simulink model "IEEE_9bus_1SG_1VSC_1DP_vol2"  (R2023b)
settings: Solver=ode8  StartTime=0.001  StopTime=60  RelTol=1e-4  EnableMultiTasking=on
PreLoadFcn:
  | ct = 1.083
values from neighbouring files (symbols this model uses):
  kp3 = 5    [main.m]
  Pmax3 = 1.15    [main.m]
  Pmin3 = 0.850    (= 0.85)    [main.m]
  Pnom = 100e6    (= 100000000)    [main.m]
  t_st = 5    [main.m]
  ts_pi = 5    [main.m]
  Vnom_prim = 230e3    (= 230000)    [main.m]
undefined symbols (not defined in the file or in its folder): D1, Delta
libraries: spsThreePhaseVIMeasurementLib x13, spsPLL3phLib x10, spsSequenceAnalyzerLib x10, spsLoadFlowBusLib x9, eeSinusoidalMeasurementV2 x9, spsThreePhasePISectionLineLib x6, slpidlib x6, jailib x4, spsPowerPositiveSequenceLib x4, spsThreePhaseTransformerTwoWindingsLib x3, spsMeanLib x3, spsDCVoltageSourceLib x2
(part 1 of 2)
settings Model: Creator=jp536285  LastModifiedBy=Administrator
settings SolverCC: AlgebraicLoopSolver=TrustRegion  AutoInsertRateTranBlk=on
settings DataIOCC: FinalStateName=xFinal_no_ex_vol2  InitialState=xFinal_no_ex_vol2  LoadInitialState=on  SaveOperatingPoint=on  SaveFormat=Array  SaveOutput=off  SaveTime=off  ReturnWorkspaceOutputs=off
settings OptimizationCC: LifeSpan=inf
settings DebuggingCC: UnderspecifiedInitializationDetection=Classic  MergeDetectMultiDrivingBlocksExec=none  SolverPrmCheckMsg=warning  StateNameClashWarn=warning  SFUnexpectedBacktrackingDiag=warning  SFNoUnconditionalDefaultTransitionDiag=warning  SFExecutionAtInitializationDiag=none  ArithmeticOperatorsInVariantConditions=warning
settings HardwareCC: ProdBitPerPointer=32  ProdBitPerSizeT=32  ProdBitPerPtrDiffT=32  ProdLargestAtomicFloat=None  ProdIntDivRoundTo=Undefined  ProdEndianess=Unspecified  ProdWordSize=32  ProdHWDeviceType=32-bit Generic
settings ModelReferenceCC: PropagateSignalLabelsOutOfModel=off
settings SFSimCC: SimUseLocalCustomCode=off  CustomCodeUndefinedFunction=UseInterfaceOnly
settings RTWCC: RTWUseLocalCustomCode=off
settings CodeAppCC: StateflowObjectComments=on
settings GRTTargetCC: TargetLangStandard=C89/C90 (ANSI)
settings ConfigComp: CovMetricSettings=dw  CovSaveCumulativeToWorkspaceVar=on  CovSaveSingleToWorkspaceVar=on  CovExternalEMLEnable=off
settings SimscapeCC: SimscapeNormalizeSystem=off

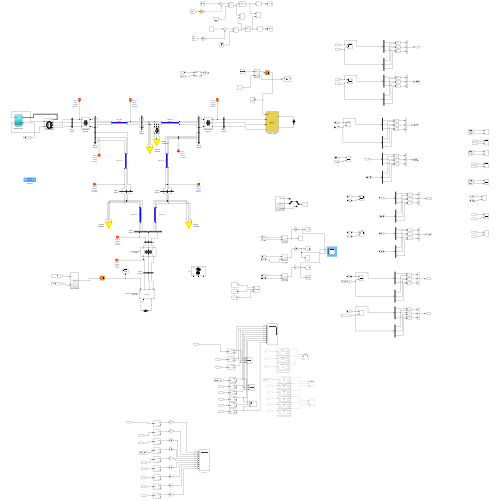
[thumbnail: Simulink's stored preview of the top-level diagram]
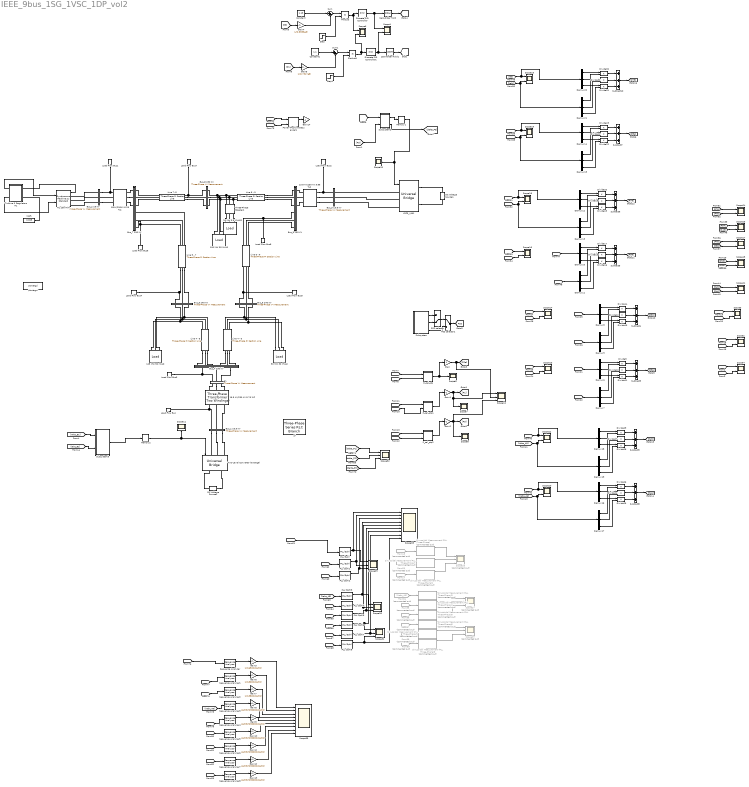
== system IEEE_9bus_1SG_1VSC_1DP_vol2 ==
  " Line 4 - 6" : spsThreePhasePISectionLineLib/Three-Phase PI Section Line  LConnTagsString=a|b|c  RConnTagsString=A|B|C  Length=100  Frequency=60  Resistances=[ 0.08993 0.224825]  Inductances="[ 1.29e-3  3.22e-3]"  Capacitances=[7.922e-9 4.74e-9]  mask(Three-Phase PI Section Line){}
      mask Display:
      | % This is a new mask on top of the base mask.
      | % Use "View base mask" link below to see the base mask.
      | patch([0.0 0.0 1 1 0.0 0.0 ],[0.4 0.7 0.7 0.4 0.4 0.7],[0 0 1]);
      | patch([0.4 0.4 0.42 0.42],[0.4 0.75 0.75 0.4],[1 0 0]);
      | patch([0.38 0.38 0.57 0.57],[0.7 0.75 0.75 0.7],[1 0 0]);
      | patch([0.53 0.53 0.55 0.55],[0.4 0.75 0.75 0.4],[1 0 0]);
  " Line 6 - 9" : spsThreePhasePISectionLineLib/Three-Phase PI Section Line  LConnTagsString=a|b|c  RConnTagsString=A|B|C  Length=100  Frequency=60  Resistances=[ 0.20631 0.5157]  Inductances="[ 2.38e-3  6.09e-3]"  Capacitances=[17.95e-9 10.55e-9]  mask(Three-Phase PI Section Line){}
      mask Display:
      | % This is a new mask on top of the base mask.
      | % Use "View base mask" link below to see the base mask.
      | patch([0.0 0.0 1 1 0.0 0.0 ],[0.4 0.7 0.7 0.4 0.4 0.7],[0 0 1]);
      | patch([0.4 0.4 0.42 0.42],[0.4 0.75 0.75 0.4],[1 0 0]);
      | patch([0.38 0.38 0.57 0.57],[0.7 0.75 0.75 0.7],[1 0 0]);
      | patch([0.53 0.53 0.55 0.55],[0.4 0.75 0.75 0.4],[1 0 0]);
  100 MW 35 MVAR : jailib/Load  SystemSampleTime=-1  VariantActivationTime=update diagram  AllowFlexibleInterface=on  Latency=0  AutoFrameSizeCalculation=off
      link override Three-Phase Parallel RLC Load: NominalVoltage=(230000)*1.01602  ActivePower=100e6  InductivePower=35e6  LoadType=constant PQ
      settings: SourceProductName=Power Library
  125 MW 50 MVAR : jailib/Load  SystemSampleTime=-1  VariantActivationTime=update diagram  AllowFlexibleInterface=on  Latency=0  AutoFrameSizeCalculation=off
      link override Three-Phase Parallel RLC Load: NominalVoltage=(230000)*0.996183  ActivePower=125e6  InductivePower=50e6  LoadType=constant PQ
      settings: SourceProductName=Power Library
  13.8 KV/230 KV 5.86 %Z : spsThreePhaseTransformerTwoWindingsLib/Three-Phase Transformer (Two Windings)  Winding1Connection=Delta (D1)  Winding2Connection=Yg  CoreType=Three single-phase transformers  SetSaturation=off  Hysteresis=off  DataFile='hysteresis'  SetInitialFlux=off  Measurements=None  UNITS=pu  NominalPower=[ 100e6 , 60 ]  Winding1=[ 13.8e3 , 1e-6 , 0 ]  Winding2=[ 230e3 , 1e-6, 0.0586 ]  Rm=500  Lm=500  L0=0.5  Saturation=[ 0,0 ; 0.0024,1.2 ; 1.0,1.52 ]  InitialFluxes=[ 0.8 , -0.8 , 0.7 ]  BreakLoop=off  DiscreteSolver=Trapezoidal iterative  DataType=off  TransfoNumber=1
  "16.5 KV/230 KV 5.76 %Z     " : spsThreePhaseTransformerTwoWindingsLib/Three-Phase Transformer (Two Windings)  Winding1Connection=Delta (D1)  Winding2Connection=Yg  CoreType=Three single-phase transformers  SetSaturation=off  Hysteresis=off  DataFile='hysteresis'  SetInitialFlux=off  Measurements=None  UNITS=pu  NominalPower=[ 100e6 , 60 ]  Winding1=[ 16.5e3 , 1e-6, 0 ]  Winding2=[ 230e3 ,1e-6, 0.0576 ]  Rm=500  Lm=500  L0=0.5  Saturation=[ 0,0 ; 0.0024,1.2 ; 1.0,1.52 ]  InitialFluxes=[ 0.8 , -0.8 , 0.7 ]  BreakLoop=off  DiscreteSolver=Trapezoidal iterative  DataType=off  TransfoNumber=1
  18KV/230KV 6.25 %Z : spsThreePhaseTransformerTwoWindingsLib/Three-Phase Transformer (Two Windings)  Winding1Connection=Delta (D1)  Winding2Connection=Yg  CoreType=Three single-phase transformers  SetSaturation=off  Hysteresis=off  DataFile='hysteresis'  SetInitialFlux=off  Measurements=None  UNITS=pu  NominalPower=[ 100e6 , 60 ]  Winding1=[ 18e3 , 1e-6 , 0]  Winding2=[ 230e3 , 1e-6, 0.0625 ]  Rm=500  Lm=500  L0=0.5  Saturation=[ 0,0 ; 0.0024,1.2 ; 1.0,1.52 ]  InitialFluxes=[ 0.8 , -0.8 , 0.7 ]  BreakLoop=off  DiscreteSolver=Trapezoidal iterative  DataType=off  TransfoNumber=1
  20 MW 3.5 MVAR2 : jailib/Load  SystemSampleTime=-1  VariantActivationTime=update diagram  AllowFlexibleInterface=on  Latency=0  AutoFrameSizeCalculation=off
      link override Three-Phase Parallel RLC Load: NominalVoltage=(230000)*1.01602  ActivePower=10e6  InductivePower=0  LoadType=constant PQ
      settings: SourceProductName=Power Library
  90 MW 30 MVAR : jailib/Load  SystemSampleTime=-1  VariantActivationTime=update diagram  AllowFlexibleInterface=on  Latency=0  AutoFrameSizeCalculation=off
      link override Three-Phase Parallel RLC Load: NominalVoltage=(230000)*1.01315  ActivePower=90e6  InductivePower=30e6  LoadType=constant PQ
      settings: SourceProductName=Power Library
  B1 : spsThreePhaseVIMeasurementLib/Three-Phase V-I Measurement  VoltageMeasurement=phase-to-ground  SetLabelV=on  LabelV=Vabc_B1  Vpu=off  VpuLL=off  CurrentMeasurement=yes  SetLabelI=on  LabelI=Iabc_B1  Ipu=off  Pbase=100e6  Vbase=500e3  OutputType=Magnitude  PhasorSimulation=off  PSBequivalent=0
  Bus_1 16.5 KV : spsThreePhaseVIMeasurementLib/Three-Phase V-I Measurement  VoltageMeasurement=phase-to-phase  SetLabelV=on  LabelV=Vabc_1  Vpu=off  VpuLL=off  CurrentMeasurement=yes  SetLabelI=on  LabelI=Iabc_1  Ipu=off  Pbase=100e6  Vbase=16.5e3  OutputType=Complex  PhasorSimulation=off  PSBequivalent=0
  Bus_2 18 KV : spsThreePhaseVIMeasurementLib/Three-Phase V-I Measurement  VoltageMeasurement=phase-to-phase  SetLabelV=on  LabelV=Vabc_2  Vpu=off  VpuLL=off  CurrentMeasurement=yes  SetLabelI=on  LabelI=Iabc_2  Ipu=off  Pbase=100e6  Vbase=18e3  OutputType=Complex  PhasorSimulation=off  PSBequivalent=0
  Bus_3 13.8 KV : spsThreePhaseVIMeasurementLib/Three-Phase V-I Measurement  VoltageMeasurement=phase-to-phase  SetLabelV=on  LabelV=Vabc_3  Vpu=off  VpuLL=off  CurrentMeasurement=yes  SetLabelI=on  LabelI=Iabc_3  Ipu=off  Pbase=100e6  Vbase=13.8e3  OutputType=Complex  PhasorSimulation=off  PSBequivalent=0
  Bus_4 230 KV : Subsystem
  Bus_5 230 KV : spsThreePhaseVIMeasurementLib/Three-Phase V-I Measurement  VoltageMeasurement=phase-to-ground  SetLabelV=on  LabelV=Vabc_5  Vpu=off  VpuLL=off  CurrentMeasurement=yes  SetLabelI=on  LabelI=Iabc_5  Ipu=off  Pbase=100e6  Vbase=230e3  OutputType=Complex  PhasorSimulation=off  PSBequivalent=0
  Bus_6 230 KV : spsThreePhaseVIMeasurementLib/Three-Phase V-I Measurement  VoltageMeasurement=phase-to-ground  SetLabelV=on  LabelV=Vabc_6  Vpu=off  VpuLL=off  CurrentMeasurement=yes  SetLabelI=on  LabelI=Iabc_6  Ipu=off  Pbase=100e6  Vbase=230e3  OutputType=Complex  PhasorSimulation=off  PSBequivalent=0
  Bus_7 230 KV : Subsystem
  Bus_8 230 KV : spsThreePhaseVIMeasurementLib/Three-Phase V-I Measurement  VoltageMeasurement=phase-to-ground  SetLabelV=on  LabelV=Vabc_8  Vpu=off  VpuLL=off  CurrentMeasurement=yes  SetLabelI=on  LabelI=Iabc_8  Ipu=off  Pbase=100e6  Vbase=230e3  OutputType=Complex  PhasorSimulation=off  PSBequivalent=0
  Bus_9 230 KV : Subsystem
  Constant : Constant  Value=1.13
  Constant1 : Constant  Value=1.1
  DC Voltage Source1 : spsDCVoltageSourceLib/DC Voltage Source  Amplitude=2*13.8e3  Measurements=None
  DC Voltage Source2 : spsDCVoltageSourceLib/DC Voltage Source  Amplitude=2*16.5e3  Measurements=None
  Demux{6..21} (16 alike) : Demux  Outputs=3
  Discrete PID Controller : slpidlib/PID Controller  Controller=PI  Form=Parallel  TimeDomain=Discrete-time  UseExternalTs=off  SampleTime=-1  IntegratorMethod=Forward Euler  FilterMethod=Forward Euler  ControllerParametersSource=internal  P=0.001  I=0.015  UseKiTs=off  D=0  N=100  UseFilter=on  TunerSelectOption=Transfer Function Based (PID Tuner App)  InitialConditionSource=internal  InitialConditionForIntegrator=0  InitialConditionForFilter=0  DifferentiatorICPrevScaledInput=0  ExternalReset=none  TrackingMode=off  Kt=1  LimitOutput=off  SatLimitsSource=internal  UpperSaturationLimit=inf  LowerSaturationLimit=-inf  LinearizeAsGain=off  AntiWindupMode=none  Kb=1  LimitIntegrator=off  UpperIntegratorSaturationLimit=inf  LowerIntegratorSaturationLimit=-inf  POutMin=[]  POutMax=[]  IOutMin=[]  IOutMax=[]  DOutMin=[]  DOutMax=[]  NOutMin=[]  NOutMax=[]  SumOutMin=[]  SumOutMax=[]  SaturationOutMin=[]  SaturationOutMax=[]  PParamMin=[]  PParamMax=[]  IParamMin=[]  IParamMax=[]  DParamMin=[]  DParamMax=[]  NParamMin=[]  NParamMax=[]  KbParamMin=[]  KbParamMax=[]  KtParamMin=[]  KtParamMax=[]  KbOutMin=[]  KbOutMax=[]  KtOutMin=[]  KtOutMax=[]  IntegratorOutMin=[]  IntegratorOutMax=[]  FilterOutMin=[]  FilterOutMax=[]  SumI1OutMin=[]  SumI1OutMax=[]  SumI2OutMin=[]  SumI2OutMax=[]  SumI3OutMin=[]  SumI3OutMax=[]  SumI4OutMin=[]  SumI4OutMax=[]  SumDOutMin=[]  SumDOutMax=[]  DifferentiatorOutMin=[]  DifferentiatorOutMax=[]  FilterDiffOutCoefMin=[]  FilterDiffOutCoefMax=[]  ReciprocalOutMin=[]  ReciprocalOutMax=[]  SumDenOutMin=[]  SumDenOutMax=[]  SumNumOutMin=[]  SumNumOutMax=[]  DivideOutMin=[]  DivideOutMax=[]  UdiffTsProdOutMin=[]  UdiffTsProdOutMax=[]  NTsProdOutMin=[]  NTsProdOutMax=[]  UintegralTsProdOutMin=[]  UintegralTsProdOutMax=[]  UngainTsProdOutMin=[]  UngainTsProdOutMax=[]  ClampingZeroOutDataTypeStr=Inherit: Inherit via back propagation  ClampingZeroOutMin=[]  ClampingZeroOutMax=[]  FilterDenConstantOutDataTypeStr=Inherit: Inherit via back propagation  FilterDenConstantOutMin=[]  FilterDenConstantOutMax=[]  PCopyOutDataTypeStr=Inherit: Inherit via back propagation  PCopyOutMin=[]  PCopyOutMax=[]  NCopyOutDataTypeStr=Inherit: Inherit via back propagation  NCopyOutMin=[]  NCopyOutMax=[]  IntegratorContinuousStateAttributes=''  IntegratorStateMustResolveToSignalObject=off  IntegratorRTWStateStorageClass=Auto  FilterContinuousStateAttributes=''  FilterStateMustResolveToSignalObject=off  FilterRTWStateStorageClass=Auto  ParallelPVariant=InternalParameters  IdealPVariant=Disabled  IVariant=InternalParameters  DVariant=Disabled  IntegratorVariant=Discrete  SatVariant=Disabled  AWVariant=Passthrough  PCopyVariant=Disabled  TRVariant=Disabled  FdbkBlocksVariant=Forward  IdealPFdbkVariant=Disabled  SatFdbkVariant=Disabled  DerivativeFilterVariant=Disabled  NVariant=Disabled  NCopyVariant=Disabled_SignalSpec  FilterICVariant=Disabled  IntegratorICVariant=InternalICs  ExternalResetVariant=Disabled  TRSumVariant=Passthrough  SumFdbkVariant=Disabled  SumVariant=Sum_PI  TsampFilterVariant=InternalTs  TsampNgainVariant=Passthrough  TsampIntegralVariant=Disabled_SignalSpec  ExternalSaturationOutDataTypeStr=Inherit: Same as second input
      settings: LibrarySourceBlock=simulink/Discrete/Discrete PID Controller
  Discrete PID Controller1 : slpidlib/PID Controller  Controller=PI  Form=Parallel  TimeDomain=Discrete-time  UseExternalTs=off  SampleTime=-1  IntegratorMethod=Forward Euler  FilterMethod=Forward Euler  ControllerParametersSource=internal  P=0.001  I=0.015  UseKiTs=off  D=0  N=100  UseFilter=on  TunerSelectOption=Transfer Function Based (PID Tuner App)  InitialConditionSource=internal  InitialConditionForIntegrator=0  InitialConditionForFilter=0  DifferentiatorICPrevScaledInput=0  ExternalReset=none  TrackingMode=off  Kt=1  LimitOutput=off  SatLimitsSource=internal  UpperSaturationLimit=inf  LowerSaturationLimit=-inf  LinearizeAsGain=off  AntiWindupMode=none  Kb=1  LimitIntegrator=off  UpperIntegratorSaturationLimit=inf  LowerIntegratorSaturationLimit=-inf  POutMin=[]  POutMax=[]  IOutMin=[]  IOutMax=[]  DOutMin=[]  DOutMax=[]  NOutMin=[]  NOutMax=[]  SumOutMin=[]  SumOutMax=[]  SaturationOutMin=[]  SaturationOutMax=[]  PParamMin=[]  PParamMax=[]  IParamMin=[]  IParamMax=[]  DParamMin=[]  DParamMax=[]  NParamMin=[]  NParamMax=[]  KbParamMin=[]  KbParamMax=[]  KtParamMin=[]  KtParamMax=[]  KbOutMin=[]  KbOutMax=[]  KtOutMin=[]  KtOutMax=[]  IntegratorOutMin=[]  IntegratorOutMax=[]  FilterOutMin=[]  FilterOutMax=[]  SumI1OutMin=[]  SumI1OutMax=[]  SumI2OutMin=[]  SumI2OutMax=[]  SumI3OutMin=[]  SumI3OutMax=[]  SumI4OutMin=[]  SumI4OutMax=[]  SumDOutMin=[]  SumDOutMax=[]  DifferentiatorOutMin=[]  DifferentiatorOutMax=[]  FilterDiffOutCoefMin=[]  FilterDiffOutCoefMax=[]  ReciprocalOutMin=[]  ReciprocalOutMax=[]  SumDenOutMin=[]  SumDenOutMax=[]  SumNumOutMin=[]  SumNumOutMax=[]  DivideOutMin=[]  DivideOutMax=[]  UdiffTsProdOutMin=[]  UdiffTsProdOutMax=[]  NTsProdOutMin=[]  NTsProdOutMax=[]  UintegralTsProdOutMin=[]  UintegralTsProdOutMax=[]  UngainTsProdOutMin=[]  UngainTsProdOutMax=[]  ClampingZeroOutDataTypeStr=Inherit: Inherit via back propagation  ClampingZeroOutMin=[]  ClampingZeroOutMax=[]  FilterDenConstantOutDataTypeStr=Inherit: Inherit via back propagation  FilterDenConstantOutMin=[]  FilterDenConstantOutMax=[]  PCopyOutDataTypeStr=Inherit: Inherit via back propagation  PCopyOutMin=[]  PCopyOutMax=[]  NCopyOutDataTypeStr=Inherit: Inherit via back propagation  NCopyOutMin=[]  NCopyOutMax=[]  IntegratorContinuousStateAttributes=''  IntegratorStateMustResolveToSignalObject=off  IntegratorRTWStateStorageClass=Auto  FilterContinuousStateAttributes=''  FilterStateMustResolveToSignalObject=off  FilterRTWStateStorageClass=Auto  ParallelPVariant=InternalParameters  IdealPVariant=Disabled  IVariant=InternalParameters  DVariant=Disabled  IntegratorVariant=Discrete  SatVariant=Disabled  AWVariant=Passthrough  PCopyVariant=Disabled  TRVariant=Disabled  FdbkBlocksVariant=Forward  IdealPFdbkVariant=Disabled  SatFdbkVariant=Disabled  DerivativeFilterVariant=Disabled  NVariant=Disabled  NCopyVariant=Disabled_SignalSpec  FilterICVariant=Disabled  IntegratorICVariant=InternalICs  ExternalResetVariant=Disabled  TRSumVariant=Passthrough  SumFdbkVariant=Disabled  SumVariant=Sum_PI  TsampFilterVariant=InternalTs  TsampNgainVariant=Passthrough  TsampIntegralVariant=Disabled_SignalSpec  ExternalSaturationOutDataTypeStr=Inherit: Same as second input
      settings: LibrarySourceBlock=simulink/Discrete/Discrete PID Controller
  Divide{9..32} (24 alike) : Product  Inputs=**
  From17 : From  Commented=on  GotoTag=Vabc_3  TagVisibility=global
  From18 : From  Commented=on  GotoTag=Vabc_1  TagVisibility=global
  From53 : From  Commented=on  GotoTag=Vabc_2  TagVisibility=global
  From54 : From  Commented=on  GotoTag=Vabc_45  TagVisibility=global
  From55 : From  Commented=on  GotoTag=Vabc_5  TagVisibility=global
  From56 : From  Commented=on  GotoTag=Vabc_6  TagVisibility=global
  From57 : From  Commented=on  GotoTag=Vabc_7  TagVisibility=global
  From58 : From  Commented=on  GotoTag=Vabc_8  TagVisibility=global
  From59 : From  Commented=on  GotoTag=Vabc_9  TagVisibility=global
  Gain : Gain
  Gain1 : Gain  Gain=-1
  Gain{8..13} (6 alike) : Gain  Gain=sqrt(3)/(230000)/sqrt(2)
  Gain14 : Gain  Gain=-1
  Gain2 : Gain  Gain=-1
  Gain3 : Gain  Gain=1/(16500)/sqrt(2)
  Gain4 : Gain  Gain=1/(0.8553e8)
  Gain5 : Gain  Gain=1/(0.7317e8)
  Gain6 : Gain  Gain=1/(18000)/sqrt(2)
  Gain7 : Gain  Gain=1/(13800)/sqrt(2)
  "Line 4 - 5 " : spsThreePhasePISectionLineLib/Three-Phase PI Section Line  LConnTagsString=a|b|c  RConnTagsString=A|B|C  Length=100  Frequency=60  Resistances=[ 0.0529 0.13225]  Inductances="[ 1.192e-3  2.38e-3]"  Capacitances=[8.82e-9 5.188e-9]  mask(Three-Phase PI Section Line){}
      mask Display:
      | % This is a new mask on top of the base mask.
      | % Use "View base mask" link below to see the base mask.
      | patch([0.0 0.0 1 1 0.0 0.0 ],[0.4 0.7 0.7 0.4 0.4 0.7],[0 0 1]);
      | patch([0.4 0.4 0.42 0.42],[0.4 0.75 0.75 0.4],[1 0 0]);
      | patch([0.38 0.38 0.57 0.57],[0.7 0.75 0.75 0.7],[1 0 0]);
      | patch([0.53 0.53 0.55 0.55],[0.4 0.75 0.75 0.4],[1 0 0]);
  "Line 5 - 7 " : spsThreePhasePISectionLineLib/Three-Phase PI Section Line  LConnTagsString=a|b|c  RConnTagsString=A|B|C  Length=100  Frequency=60  Resistances=[ 0.16928 0.4232]  Inductances="[ 2.259e-3  5.64e-3]"  Capacitances=[15.34e-9 9.025e-9]  mask(Three-Phase PI Section Line){}
      mask Display:
      | % This is a new mask on top of the base mask.
      | % Use "View base mask" link below to see the base mask.
      | patch([0.0 0.0 1 1 0.0 0.0 ],[0.4 0.7 0.7 0.4 0.4 0.7],[0 0 1]);
      | patch([0.4 0.4 0.42 0.42],[0.4 0.75 0.75 0.4],[1 0 0]);
      | patch([0.38 0.38 0.57 0.57],[0.7 0.75 0.75 0.7],[1 0 0]);
      | patch([0.53 0.53 0.55 0.55],[0.4 0.75 0.75 0.4],[1 0 0]);
  Line 7- 8 : spsThreePhasePISectionLineLib/Three-Phase PI Section Line  LConnTagsString=a|b|c  RConnTagsString=A|B|C  Length=100  Frequency=60  Resistances=[0.044965 0.11241]  Inductances="[ 1.01e-3  2.02e-3]"  Capacitances=[7.471e-9 4.394e-9]  mask(Three-Phase PI Section Line){}
      mask Display:
      | % This is a new mask on top of the base mask.
      | % Use "View base mask" link below to see the base mask.
      | patch([0.0 0.0 1 1 0.0 0.0 ],[0.4 0.7 0.7 0.4 0.4 0.7],[0 0 1]);
      | patch([0.4 0.4 0.42 0.42],[0.4 0.75 0.75 0.4],[1 0 0]);
      | patch([0.38 0.38 0.57 0.57],[0.7 0.75 0.75 0.7],[1 0 0]);
      | patch([0.53 0.53 0.55 0.55],[0.4 0.75 0.75 0.4],[1 0 0]);
  Line 8 - 9 : spsThreePhasePISectionLineLib/Three-Phase PI Section Line  LConnTagsString=a|b|c  RConnTagsString=A|B|C  Length=100  Frequency=60  Resistances=[ 0.062951 0.15737]  Inductances="[ 1.414e-3  3.53e-3]"  Capacitances=[10.47e-9 6.15e-9]  mask(Three-Phase PI Section Line){}
      mask Display:
      | % This is a new mask on top of the base mask.
      | % Use "View base mask" link below to see the base mask.
      | patch([0.0 0.0 1 1 0.0 0.0 ],[0.4 0.7 0.7 0.4 0.4 0.7],[0 0 1]);
      | patch([0.4 0.4 0.42 0.42],[0.4 0.75 0.75 0.4],[1 0 0]);
      | patch([0.38 0.38 0.57 0.57],[0.7 0.75 0.75 0.7],[1 0 0]);
      | patch([0.53 0.53 0.55 0.55],[0.4 0.75 0.75 0.4],[1 0 0]);
  Load Flow Bus : spsLoadFlowBusLib/Load Flow Bus  LConnTagsString=a  Phases=single  Connectors=on one side  ID=BUS_1  Vbase=16.5e3  Vref=1.04  Vangle=0  VLF=1.04  VLFb=1  VLFc=1  angleLF=0  angleLFb=0  angleLFc=0
      settings: AttributesFormatString=%<ID>\n%<Vbase>V\n%<VLF>pu\n%<angleLF>deg.
  Load Flow Bus1 : spsLoadFlowBusLib/Load Flow Bus  LConnTagsString=a  Phases=single  Connectors=on one side  ID=BUS_2  Vbase=18e3  Vref=1.025  Vangle=0  VLF=1.025  VLFb=1  VLFc=1  angleLF=9.166  angleLFb=0  angleLFc=0
      settings: AttributesFormatString=%<ID>\n%<Vbase>V\n%<VLF>pu\n%<angleLF>deg.
  Load Flow Bus2 : spsLoadFlowBusLib/Load Flow Bus  LConnTagsString=a  Phases=single  Connectors=on one side  ID=BUS_3  Vbase=13.8e3  Vref=1.025  Vangle=0  VLF=1.025  VLFb=1  VLFc=1  angleLF=4.553  angleLFb=0  angleLFc=0
      settings: AttributesFormatString=%<ID>\n%<Vbase>V\n%<VLF>pu\n%<angleLF>deg.
  Load Flow Bus3 : spsLoadFlowBusLib/Load Flow Bus  LConnTagsString=a  Phases=single  Connectors=on one side  ID=BUS_4  Vbase=230e3  Vref=1  Vangle=0  VLF=1.026  VLFb=1  VLFc=1  angleLF=27.77  angleLFb=0  angleLFc=0
      settings: AttributesFormatString=%<ID>\n%<Vbase>V\n%<VLF>pu\n%<angleLF>deg.
  Load Flow Bus4 : spsLoadFlowBusLib/Load Flow Bus  LConnTagsString=a  Phases=single  Connectors=on one side  ID=BUS_5  Vbase=230e3  Vref=1  Vangle=0  VLF=0.9962  VLFb=1  VLFc=1  angleLF=25.99  angleLFb=0  angleLFc=0
      settings: AttributesFormatString=%<ID>\n%<Vbase>V\n%<VLF>pu\n%<angleLF>deg.
  Load Flow Bus5 : spsLoadFlowBusLib/Load Flow Bus  LConnTagsString=a  Phases=single  Connectors=on one side  ID=BUS_6  Vbase=230e3  Vref=1  Vangle=0  VLF=1.013  VLFb=1  VLFc=1  angleLF=26.3  angleLFb=0  angleLFc=0
      settings: AttributesFormatString=%<ID>\n%<Vbase>V\n%<VLF>pu\n%<angleLF>deg.
  Load Flow Bus6 : spsLoadFlowBusLib/Load Flow Bus  LConnTagsString=a  Phases=single  Connectors=on one side  ID=BUS_7  Vbase=230e3  Vref=1  Vangle=0  VLF=1.026  VLFb=1  VLFc=1  angleLF=33.61  angleLFb=0  angleLFc=0
      settings: AttributesFormatString=%<ID>\n%<Vbase>V\n%<VLF>pu\n%<angleLF>deg.
  Load Flow Bus7 : spsLoadFlowBusLib/Load Flow Bus  LConnTagsString=a  Phases=single  Connectors=on one side  ID=BUS_8  Vbase=230e3  Vref=1  Vangle=0  VLF=1.016  VLFb=1  VLFc=1  angleLF=30.63  angleLFb=0  angleLFc=0
      settings: AttributesFormatString=%<ID>\n%<Vbase>V\n%<VLF>pu\n%<angleLF>deg.
  Load Flow Bus8 : spsLoadFlowBusLib/Load Flow Bus  LConnTagsString=a  Phases=single  Connectors=on one side  ID=BUS_9  Vbase=230e3  Vref=1  Vangle=0  VLF=1.032  VLFb=1  VLFc=1  angleLF=31.86  angleLFb=0  angleLFc=0
      settings: AttributesFormatString=%<ID>\n%<Vbase>V\n%<VLF>pu\n%<angleLF>deg.
  M1 200 MVA : spsSynchronousMachinepuStandardLib/Synchronous Machine pu Standard  PresetModel=No  MechanicalLoad=Mechanical power Pm  ShowDetailedParameters=on  RotorType=Salient-pole  Units=per unit standard parameters  MeasurementBus=off  NominalParameters="[200E6  18000   60 ]"  Reactances1=[ 31 32 33 34 35 36 37 ]  Reactances2=[ 1.305, 0.296, 0.252, 0.474, 0.243, 0.18 ]  dAxisTimeConstants=Short-circuit  qAxisTimeConstants=Open-circuit  TimeConstants1=[]  TimeConstants2=[]  TimeConstants3=[]  TimeConstants4=[]  TimeConstants5=[ 1.01, 0.053, 0.1 ]  TimeConstants6=[]  TimeConstants7=[]  TimeConstants8=[]  StatorResistance=2.8544e-3  Mechanical="[ 3.7 0  32]"  PolePairs=32  InitialConditions=[0 -66.0372 0.836682 0.836682 0.836682 -5.70736 -125.707 114.293 1.48174]  SetSaturation=off  Saturation=[0.6404,0.7127,0.8441,0.9214,0.9956,1.082,1.19,1.316,1.457;0.7,0.7698,0.8872,0.9466,0.9969,1.046,1.1,1.151,1.201]  LoadFlowParameters=[1 950000000 0 0]  TsPowergui=0  TsBlock=-1  IterativeModel=Trapezoidal non iterative  IterativeDiscreteModel=Trapezoidal non iterative  BusType=PV  Pref=165e6  Qref=0  Qmin=-Inf  Qmax=Inf  PLF=0  QLF=0
  Memory1 : Memory
  Memory2 : Memory
  PLL (3ph){,1..8} (9 alike) : spsPLL3phLib/PLL (3ph)  Fmin=45  Par_Init=[0, 60]  ParK=[180, 3200, 1]  TcD=1e-4  MaxRateChangeFreq=200  FilterCutOffFreq=25  Ts=0  AGC=on
  PSS selector : ManualSwitch  CurrentSetting=0
  PSS selector1 : ManualSwitch
  P_cal_ptp : Subsystem
  P_cal_ptp1 : Subsystem
  P_cal_ptp2 : Subsystem
  Power (Positive-Sequence)1 : spsPowerPositiveSequenceLib/Power (Positive-Sequence)  Freq=60  Vinit=[0, 0]  Iinit=[0, 0]  Ts=1e-4
  Product : Product
  Product1 : Product
  Scope{1..4,6,13..25} (18 alike) : Scope  NumInputPorts=2
  Scope{5,7..8,10..11} (5 alike) : Scope
  Scope{12,29..32} (5 alike) : Scope  NumInputPorts=3
  Scope26 : Scope  Commented=on  NumInputPorts=3
  Scope27 : Scope  Commented=on  NumInputPorts=3
  Scope28 : Scope  Commented=on  NumInputPorts=3
  Scope33 : Scope  NumInputPorts=9
  Scope35 : Scope  NumInputPorts=9
  Sequence Analyzer{,1..8} (9 alike) : spsSequenceAnalyzerLib/Sequence Analyzer  Freq=60  n=1  seq=Positive  InInit=[1, 0]  Ts=0
      settings: LibrarySourceBlock=sps_lib/Sensors and Measurements/Sequence Analyzer
  Sinusoidal Measurement (PLL, Three-Phase){,1..8} (9 alike) : eeSinusoidalMeasurementV2/Sinusoidal Measurement (PLL, Three-Phase)  Commented=on  Kp_LF=200  Ki_LF=2000  F0=60  Theta0=0  Ts=-1
      settings: LibrarySourceBlock=|
      | ee_sl_lib/Measurements/Sinusoidal Measurement
      | (PLL, Three-Phase)
  Step : Step  Time=200  SampleTime=0
  Step1 : Step  Time=200  SampleTime=0
  Subsystem : Subsystem
  Subsystem2 : Subsystem
  Subsystem3 : Subsystem
  Subtract{3..10} (8 alike) : Sum  Inputs=+++
  Sum : Sum  Inputs=|+-
  Sum1 : Sum  Inputs=|+-
  Three-Phase Breaker1 : spsThreePhaseBreakerLib/Three-Phase Breaker  InitialState=open  SwitchA=on  SwitchB=on  SwitchC=on  SwitchTimes=[21 ]  External=off  BreakerResistance=0.001  SnubberResistance=1e7  SnubberCapacitance=inf  Measurements=None
  Turbine & Regulators M1 : Subsystem
  Two-Level Converter (average) : spsUniversalBridgeLib/Universal Bridge  Arms=3  SnubberResistance=1e5  SnubberCapacitance=inf  Device=Average-model based VSC  Ron=1e-3  Lon=0  ForwardVoltages="[  0  0  ]"  ForwardVoltage=0  GTOparameters=[ 10e-6 , 20e-6 ]  IGBTparameters=[ 1e-6 , 2e-6 ]  Measurements=None  Measurements_2=None  converterType=Rectifier
  VSC3_V/Θ1 : spsUniversalBridgeLib/Universal Bridge  Arms=3  SnubberResistance=1e5  SnubberCapacitance=inf  Device=Average-model based VSC  Ron=1e-3  Lon=0  ForwardVoltages="[  0  0  ]"  ForwardVoltage=0  GTOparameters=[ 10e-6 , 20e-6 ]  IGBTparameters=[ 1e-6 , 2e-6 ]  Measurements=None  Measurements_2=None  converterType=Rectifier
  Vref1 : Constant  Value=0.825
  Xf : spsThreePhaseSeriesRLCBranchLib/Three-Phase Series RLC Branch  LConnTagsString=A|B|C  RConnTagsString=A|B|C  BranchType=RL  Resistance=0.00005  Inductance=0.005/120/pi  Capacitance=1e-6  Measurements=None
  Zero-Order Hold : ZeroOrderHold  SampleTime=ts_pi
  Zero-Order Hold1 : ZeroOrderHold  SampleTime=ts_pi
  powergui : sps_lib/powergui  Priority=1  SimulationMode=Discrete  SampleTime=5e-5  frequency=60  Iterations=50  frequencyindice=0  Pbase=10e7  ErrMax=1e-05  UnitsV=kV  UnitsW=MW  buscounter=0  FunctionMessages=off  echomessages=off  EnableUseOfTLC=off  CurrentSourceSwitches=off  DisableSnubberDevices=off  DisableRonSwitches=off  DisableVfSwitches=off  DisplayEquations=off  AutomaticDiscreteSolvers=off  SolverType=Backward Euler  Interpol=off  ExternalGateDelay=off  methode=off  Ts=0  x0status=blocks  SPID=off  SwTol=0  HookPort=off  NonlinearTolerance=1e-4  nMaxIteration=100  ContinueOnMaxIteration=off  RestoreLinks=warning  ResistiveCurrentMeasurement=off  Frange=[0:2:500]  Ylog=off  Xlog=on  ShowGrid=off  save=off  variable=ZData  structure=0  ZoomFFT=off  StartTime=0.0  cycles=1  DisplayStyle=1  fundamental=60  FreqAxis=off  MaxFrequency=1000  frequencyindicesteady=1  RmsSteady=1  display=off
  tag scope: PSS=global
  wires:
  Demux21/3 -> Divide31/2
  Demux21/1 -> Divide32/2
  Divide30/1 -> Subtract10/2
  [Vab] -> Demux21/1, Scope23/2
  [Iab] -> Demux20/1, Scope23/1
  Subtract10/1 -> [P75]
  Demux20/2 -> Divide30/1
  Demux21/2 -> Divide30/2
  Divide32/1 -> Subtract10/1
  [Vabc_8] -> Demux11/1
  Demux15/3 -> Divide22/2
  Divide23/1 -> Subtract7/1
  Demux15/2 -> Divide21/2
  Demux14/1 -> Divide23/1
  Demux15/1 -> Divide23/2
  Subtract7/1 -> [P54]
  [Vabc_5] -> Demux15/1, Scope19/2
  Divide22/1 -> Subtract7/3
  Demux14/2 -> Divide21/1
  [Iabc_8] -> Demux10/1
  [Iabc_9] -> Scope14/1
  Demux10/1 -> Divide17/1
  [Vabc_6] -> Demux7/1
  Demux12/2 -> Divide18/1
  Demux10/2 -> Divide15/1
  Demux12/1 -> Divide20/1
  Demux8/1 -> Divide14/1
  Demux20/3 -> Divide31/1
  Subtract5/1 -> [P98]
  [Iabc_6] -> Scope13/1
  Divide20/1 -> Subtract6/1
  Demux12/3 -> Divide19/1
  Divide17/1 -> Subtract5/1
  Demux7/2 -> Divide10/2
  Subtract6/1 -> [P78]
  [Vabc_7] -> Demux13/1, Scope18/2
  Demux10/3 -> Divide16/1
  [Iabc_7] -> Demux12/1, Scope18/1
  Demux11/1 -> Divide17/2
  Demux7/1 -> Divide9/2
  Demux13/3 -> Divide19/2
  Demux9/2 -> Divide12/2
  Divide19/1 -> Subtract6/3
  [Vabc_9] -> Demux9/1
  Divide16/1 -> Subtract5/3
  [Vabc_8] -> Scope16/2
  Divide18/1 -> Subtract6/2
  Divide14/1 -> Subtract4/1
  Divide13/1 -> Subtract4/3
  Divide10/1 -> Subtract3/2
  Demux8/2 -> Divide12/1
  [Iabc_9] -> Demux8/1
  Demux6/3 -> Divide11/1
  [Vabc_9] -> Scope14/2
  Divide9/1 -> Subtract3/1
  [Vabc_6] -> Scope13/2
  Demux8/3 -> Divide13/1
  Divide15/1 -> Subtract5/2
  Divide11/1 -> Subtract3/3
  [Iabc_46] -> Demux16/1, Scope20/1
  Demux13/1 -> Divide20/2
  Demux17/3 -> Divide25/2
  [Vabc_46] -> Demux17/1, Scope20/2
  [Iabc_8] -> Scope16/1
  Demux13/2 -> Divide18/2
  Demux17/2 -> Divide24/2
  Demux6/2 -> Divide10/1
  Demux9/1 -> Divide14/2
  Divide28/1 -> Subtract9/3
  Demux16/3 -> Divide25/1
  Subtract3/1 -> [P96]
  Demux19/3 -> Divide28/2
  Demux17/1 -> Divide26/2
  Divide12/1 -> Subtract4/2
  Demux7/3 -> Divide11/2
  Divide27/1 -> Subtract9/2
  Demux6/1 -> Divide9/1
  [Iabc_45] -> Demux18/1, Scope22/1
  Demux9/3 -> Divide13/2
  [Vabc_45] -> Scope22/2, Demux19/1
  Demux19/1 -> Divide29/2
  Divide21/1 -> Subtract7/2
  Demux11/3 -> Divide16/2
  Divide24/1 -> Subtract8/2
  [Iabc_6] -> Demux6/1
  Subtract9/1 -> [P45]
  Divide31/1 -> Subtract10/3
  Divide29/1 -> Subtract9/1
  Divide25/1 -> Subtract8/3
  Demux16/1 -> Divide26/1
  Demux14/3 -> Divide22/1
  Demux16/2 -> Divide24/1
  Demux19/2 -> Divide27/2
  Demux11/2 -> Divide15/2
  Demux18/2 -> Divide27/1
  Demux18/1 -> Divide29/1
  Demux20/1 -> Divide32/1
  Subtract4/1 -> [P93]
  Demux18/3 -> Divide28/1
  Subtract8/1 -> [P46]
  [Iabc_5] -> Demux14/1, Scope19/1
  Divide26/1 -> Subtract8/1
  [P78] -> Scope24/2
  [P93] -> Scope15/1
  [P75] -> Scope24/1
  [P46] -> Scope21/2
  [P45] -> Scope21/1
  [P45] -> Scope25/2
  [P78] -> Scope17/1
  [Vabc_3] -> Scope3/2
  [P96] -> Scope15/2
  [Iabc_2] -> Scope2/1
  [Iabc_1] -> Scope4/1
  [Iabc_3] -> Scope3/1
  [P54] -> Scope25/1
  [P98] -> Scope17/2
  [Vabc_1] -> Scope4/2
  [Vabc_2] -> Scope2/2
  [Iabc_2] -> P_cal_ptp/1(In1)
  [Vabc_2] -> P_cal_ptp/2(In2)
  Gain/1 -> Scope12/2, [P2e]
  [Iabc_1] -> P_cal_ptp1/1(In1)
  P_cal_ptp1/1(Out1) -> Gain1/1
  Gain1/1 -> Scope12/1, Scope7/1, [P1]
  [Iabc_3] -> P_cal_ptp2/1(In1)
  [Vabc_3] -> P_cal_ptp2/2(In2)
  P_cal_ptp2/1(Out1) -> Gain2/1
  Gain2/1 -> Scope12/3, Scope8/1, [P3]
  Subsystem2/1(Out1) -> Memory1/1
  Memory1/1 -> Scope10/1, VSC3_V/Θ1/1
  Subsystem3/1(Uabc_ref) -> Memory2/1
  Memory2/1 -> Two-Level Converter (average)/1, Scope11/1
  Step/1 -> Product/2
  Step1/1 -> Product1/2
  [delta3] -> Subsystem2/1(delta)
  [P3] -> Gain4/1
  Constant/1 -> Sum/1
  [P1] -> Gain5/1
  Constant1/1 -> Sum1/1
  Gain4/1 -> Sum/2
  Gain5/1 -> Sum1/2
  Product/1 -> Scope6/1, Discrete PID Controller/1
  Sum/1 -> Product/1
  Discrete PID Controller/1 -> Zero-Order Hold/1, Scope1/1
  Sum1/1 -> Product1/1
  Product1/1 -> Discrete PID Controller1/1, Scope6/2
  Discrete PID Controller1/1 -> Zero-Order Hold1/1, Scope1/2
  P_cal_ptp/1(Out1) -> Gain/1, Scope5/1
  Zero-Order Hold/1 -> [delta3]
  Zero-Order Hold1/1 -> [delta1]
  From17/1 -> "Sinusoidal Measurement (PLL, Three-Phase)2"/1
  From18/1 -> "Sinusoidal Measurement (PLL, Three-Phase)"/1
  From53/1 -> "Sinusoidal Measurement (PLL, Three-Phase)1"/1
  From54/1 -> "Sinusoidal Measurement (PLL, Three-Phase)3"/1
  From55/1 -> "Sinusoidal Measurement (PLL, Three-Phase)4"/1
  From56/1 -> "Sinusoidal Measurement (PLL, Three-Phase)5"/1
  From57/1 -> "Sinusoidal Measurement (PLL, Three-Phase)6"/1
  From58/1 -> "Sinusoidal Measurement (PLL, Three-Phase)7"/1
  From59/1 -> "Sinusoidal Measurement (PLL, Three-Phase)8"/1
  "Sinusoidal Measurement (PLL, Three-Phase)"/1 -> Scope26/1
  "Sinusoidal Measurement (PLL, Three-Phase)1"/1 -> Scope26/2
  "Sinusoidal Measurement (PLL, Three-Phase)2"/1 -> Scope26/3
  "Sinusoidal Measurement (PLL, Three-Phase)3"/1 -> Scope27/1
  "Sinusoidal Measurement (PLL, Three-Phase)4"/1 -> Scope27/2
  "Sinusoidal Measurement (PLL, Three-Phase)5"/1 -> Scope27/3
  "Sinusoidal Measurement (PLL, Three-Phase)6"/1 -> Scope28/1
  "Sinusoidal Measurement (PLL, Three-Phase)7"/1 -> Scope28/2
  "Sinusoidal Measurement (PLL, Three-Phase)8"/1 -> Scope28/3
  [Vabc_7] -> PLL (3ph)6/1
  [Vabc_45] -> PLL (3ph)3/1
  [Vabc_2] -> PLL (3ph)1/1
  [Vabc_8] -> PLL (3ph)7/1
  [Vabc_9] -> PLL (3ph)8/1
  [Vabc_5] -> PLL (3ph)4/1
  [Vabc_3] -> PLL (3ph)2/1
  [Vabc_6] -> PLL (3ph)5/1
  PLL (3ph)/1 -> Scope33/1, Scope29/1
  PLL (3ph)1/1 -> Scope33/2, Scope29/2
  PLL (3ph)2/1 -> Scope33/3, Scope29/3
  PLL (3ph)4/1 -> Scope33/5, Scope30/2
  PLL (3ph)3/1 -> Scope33/4, Scope30/1
  PLL (3ph)5/1 -> Scope33/6, Scope30/3
  PLL (3ph)7/1 -> Scope31/2, Scope33/8
  PLL (3ph)6/1 -> Scope33/7, Scope31/1
  PLL (3ph)8/1 -> Scope33/9, Scope31/3
  Subsystem2/2(Out4) -> [delta_P3]
  [delta_P1] -> Scope32/1
  [delta_P2] -> Scope32/2
  [delta_P3] -> Scope32/3
  [Vabc_8] -> Sequence Analyzer7/1
  [Vabc_7] -> Sequence Analyzer6/1
  [Vabc_2] -> Sequence Analyzer1/1
  [Vabc_45] -> Sequence Analyzer3/1
  [Vabc_9] -> Sequence Analyzer8/1
  [Vabc_3] -> Sequence Analyzer2/1
  [Vabc_5] -> Sequence Analyzer4/1
  [Vabc_6] -> Sequence Analyzer5/1
  Sequence Analyzer/1 -> Gain3/1
  Sequence Analyzer1/1 -> Gain6/1
  Sequence Analyzer2/1 -> Gain7/1
  Sequence Analyzer3/1 -> Gain8/1
  Sequence Analyzer4/1 -> Gain9/1
  Sequence Analyzer5/1 -> Gain10/1
  Sequence Analyzer6/1 -> Gain11/1
  Sequence Analyzer7/1 -> Gain12/1
  Sequence Analyzer8/1 -> Gain13/1
  Gain3/1 -> Scope35/1
  Gain6/1 -> Scope35/2
  Gain7/1 -> Scope35/3
  Gain8/1 -> Scope35/4
  Gain9/1 -> Scope35/5
  Gain10/1 -> Scope35/6
  Gain11/1 -> Scope35/7
  Gain12/1 -> Scope35/8
  Gain13/1 -> Scope35/9
  [Vabc_1] -> Sequence Analyzer/1
  [Vabc_1] -> PLL (3ph)/1
  [Vabc_1] -> P_cal_ptp1/2(In2)
  Turbine & Regulators M1/1(Pm) -> M1 200 MVA/1
  [Vabc_B1] -> Subsystem3/1(V)
  [Iabc_B1] -> Subsystem3/2(I)
  [Iabc_9] -> Power (Positive-Sequence)1/1
  [Vabc_9] -> Power (Positive-Sequence)1/2
  Power (Positive-Sequence)1/1 -> Gain14/1
  [P3] -> Subsystem2/2(P3)
  Vref1/1 -> Turbine & Regulators M1/2(Pref)
  M1 200 MVA/1 -> Turbine & Regulators M1/1(m)
  Turbine & Regulators M1/2(Vf) -> M1 200 MVA/2
  Subsystem/1(Generic) -> PSS selector/1
  PSS selector1/1 -> [PSS]
  Subsystem/2(Multiband) -> PSS selector/2
  PSS selector/1 -> PSS selector1/1
  Subsystem/3(No PSS) -> PSS selector1/2
  connections:
  18KV/230KV 6.25 %Z/LConn2 -- Bus_2 18 KV/RConn2
  18KV/230KV 6.25 %Z/RConn2 -- Bus_7 230 KV/LConn2
  Bus_2 18 KV/RConn1 -- Load Flow Bus1/LConn1 -- 18KV/230KV 6.25 %Z/LConn1
  Bus_2 18 KV/RConn3 -- 18KV/230KV 6.25 %Z/LConn3
  Bus_7 230 KV/LConn1 -- 18KV/230KV 6.25 %Z/RConn1
  18KV/230KV 6.25 %Z/RConn3 -- Bus_7 230 KV/LConn3
  13.8 KV/230 KV 5.86 %Z/LConn1 -- Bus_3 13.8 KV/LConn1 -- Load Flow Bus2/LConn1
  13.8 KV/230 KV 5.86 %Z/LConn2 -- Bus_3 13.8 KV/LConn2
  13.8 KV/230 KV 5.86 %Z/LConn3 -- Bus_3 13.8 KV/LConn3
  Bus_1 16.5 KV/LConn3 -- "16.5 KV/230 KV 5.76 %Z     "/LConn3
  Bus_1 16.5 KV/LConn2 -- "16.5 KV/230 KV 5.76 %Z     "/LConn2
  13.8 KV/230 KV 5.86 %Z/RConn1 -- Bus_9 230 KV/RConn1
  13.8 KV/230 KV 5.86 %Z/RConn2 -- Bus_9 230 KV/RConn2
  13.8 KV/230 KV 5.86 %Z/RConn3 -- Bus_9 230 KV/RConn3
  Load Flow Bus3/LConn1 -- B1/RConn1 -- Bus_4 230 KV/LConn1
  Line 8 - 9/LConn1 -- Three-Phase Breaker1/LConn1 -- Bus_8 230 KV/LConn1 -- 100 MW 35 MVAR/LConn1
  Line 8 - 9/LConn2 -- Three-Phase Breaker1/LConn2 -- Bus_8 230 KV/LConn2 -- 100 MW 35 MVAR/LConn2
  Line 8 - 9/LConn3 -- Three-Phase Breaker1/LConn3 -- 100 MW 35 MVAR/LConn3 -- Bus_8 230 KV/LConn3
  "Line 4 - 5 "/LConn1 -- 125 MW 50 MVAR/LConn1 -- Bus_5 230 KV/RConn1
  "Line 4 - 5 "/LConn2 -- 125 MW 50 MVAR/LConn2 -- Bus_5 230 KV/RConn2
  "Line 4 - 5 "/LConn3 -- 125 MW 50 MVAR/LConn3 -- Bus_5 230 KV/RConn3
  " Line 4 - 6"/LConn1 -- 90 MW 30 MVAR/LConn1 -- Bus_6 230 KV/RConn1
  " Line 4 - 6"/LConn2 -- 90 MW 30 MVAR/LConn2 -- Bus_6 230 KV/RConn2
  " Line 4 - 6"/LConn3 -- 90 MW 30 MVAR/LConn3 -- Bus_6 230 KV/RConn3
  Line 7- 8/LConn1 -- Bus_7 230 KV/RConn1
  Line 7- 8/LConn2 -- Bus_7 230 KV/RConn2
  Bus_7 230 KV/RConn3 -- Line 7- 8/LConn3
  Bus_8 230 KV/RConn1 -- Line 7- 8/RConn1 -- Load Flow Bus7/LConn1
  Line 7- 8/RConn2 -- Bus_8 230 KV/RConn2
  Line 7- 8/RConn3 -- Bus_8 230 KV/RConn3
  Line 8 - 9/RConn2 -- Bus_9 230 KV/LConn2
  Line 8 - 9/RConn1 -- Bus_9 230 KV/LConn1
  Line 8 - 9/RConn3 -- Bus_9 230 KV/LConn3
  " Line 6 - 9"/RConn1 -- Load Flow Bus8/LConn1 -- Bus_9 230 KV/LConn4
  Bus_9 230 KV/LConn5 -- " Line 6 - 9"/RConn2
  Bus_6 230 KV/LConn1 -- " Line 6 - 9"/LConn1 -- Load Flow Bus5/LConn1
  Bus_6 230 KV/LConn2 -- " Line 6 - 9"/LConn2
  Bus_6 230 KV/LConn3 -- " Line 6 - 9"/LConn3
  " Line 6 - 9"/RConn3 -- Bus_9 230 KV/LConn6
  "Line 4 - 5 "/RConn2 -- Bus_4 230 KV/RConn2
  "Line 4 - 5 "/RConn1 -- Bus_4 230 KV/RConn1
  "Line 4 - 5 "/RConn3 -- Bus_4 230 KV/RConn3
  " Line 4 - 6"/RConn2 -- Bus_4 230 KV/RConn5
  " Line 4 - 6"/RConn1 -- Bus_4 230 KV/RConn4
  " Line 4 - 6"/RConn3 -- Bus_4 230 KV/RConn6
  Bus_1 16.5 KV/LConn1 -- "16.5 KV/230 KV 5.76 %Z     "/LConn1 -- Load Flow Bus/LConn1
  Bus_7 230 KV/RConn6 -- "Line 5 - 7 "/LConn1 -- Load Flow Bus6/LConn1
  Load Flow Bus4/LConn1 -- "Line 5 - 7 "/RConn1 -- Bus_5 230 KV/LConn1
  VSC3_V/Θ1/LConn2 -- Bus_3 13.8 KV/RConn2
  VSC3_V/Θ1/LConn1 -- Bus_3 13.8 KV/RConn1
  VSC3_V/Θ1/LConn3 -- Bus_3 13.8 KV/RConn3
  VSC3_V/Θ1/RConn2 -- DC Voltage Source1/LConn1
  VSC3_V/Θ1/RConn1 -- DC Voltage Source1/RConn1
  Two-Level Converter (average)/RConn1 -- DC Voltage Source2/RConn1
  DC Voltage Source2/LConn1 -- Two-Level Converter (average)/RConn2
  "Line 5 - 7 "/RConn2 -- Bus_5 230 KV/LConn2
  "Line 5 - 7 "/RConn3 -- Bus_5 230 KV/LConn3
  "Line 5 - 7 "/LConn2 -- Bus_7 230 KV/RConn5
  "Line 5 - 7 "/LConn3 -- Bus_7 230 KV/RConn4
  20 MW 3.5 MVAR2/LConn2 -- Three-Phase Breaker1/RConn2
  20 MW 3.5 MVAR2/LConn1 -- Three-Phase Breaker1/RConn1
  20 MW 3.5 MVAR2/LConn3 -- Three-Phase Breaker1/RConn3
  Bus_2 18 KV/LConn2 -- M1 200 MVA/RConn2
  Bus_2 18 KV/LConn3 -- M1 200 MVA/RConn3
  Bus_2 18 KV/LConn1 -- M1 200 MVA/RConn1
  Bus_1 16.5 KV/RConn2 -- Two-Level Converter (average)/LConn2
  Bus_1 16.5 KV/RConn3 -- Two-Level Converter (average)/LConn3
  Bus_1 16.5 KV/RConn1 -- Two-Level Converter (average)/LConn1
  Bus_4 230 KV/LConn3 -- B1/RConn3
  B1/RConn2 -- Bus_4 230 KV/LConn2
  B1/LConn1 -- "16.5 KV/230 KV 5.76 %Z     "/RConn1
  B1/LConn2 -- "16.5 KV/230 KV 5.76 %Z     "/RConn2
  B1/LConn3 -- "16.5 KV/230 KV 5.76 %Z     "/RConn3

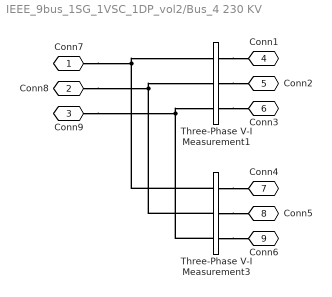
== system IEEE_9bus_1SG_1VSC_1DP_vol2/Bus_4 230 KV ==
  Three-Phase V-I Measurement1 : spsThreePhaseVIMeasurementLib/Three-Phase V-I Measurement  VoltageMeasurement=phase-to-ground  SetLabelV=on  LabelV=Vabc_45  Vpu=off  VpuLL=off  CurrentMeasurement=yes  SetLabelI=on  LabelI=Iabc_45  Ipu=off  Pbase=100e6  Vbase=230e3  OutputType=Complex  PhasorSimulation=off  PSBequivalent=0
  Three-Phase V-I Measurement3 : spsThreePhaseVIMeasurementLib/Three-Phase V-I Measurement  VoltageMeasurement=phase-to-ground  SetLabelV=on  LabelV=Vabc_46  Vpu=off  VpuLL=off  CurrentMeasurement=yes  SetLabelI=on  LabelI=Iabc_46  Ipu=off  Pbase=100e6  Vbase=230e3  OutputType=Complex  PhasorSimulation=off  PSBequivalent=0
  Conn7 : PMIOPort  Side=Left
  Conn8 : PMIOPort  Port=2  Side=Left
  Conn9 : PMIOPort  Port=3  Side=Left
  Conn1 : PMIOPort  Port=4  Side=Right
  Conn2 : PMIOPort  Port=5  Side=Right
  Conn3 : PMIOPort  Port=6  Side=Right
  Conn4 : PMIOPort  Port=7  Side=Right
  Conn5 : PMIOPort  Port=8  Side=Right
  Conn6 : PMIOPort  Port=9  Side=Right
  connections:
  Three-Phase V-I Measurement3/LConn3 -- Conn9/RConn1 -- Three-Phase V-I Measurement1/LConn3
  Three-Phase V-I Measurement3/LConn2 -- Conn8/RConn1 -- Three-Phase V-I Measurement1/LConn2
  Three-Phase V-I Measurement3/LConn1 -- Conn7/RConn1 -- Three-Phase V-I Measurement1/LConn1
  Three-Phase V-I Measurement3/RConn3 -- Conn6/RConn1
  Three-Phase V-I Measurement1/RConn3 -- Conn3/RConn1
  Three-Phase V-I Measurement1/RConn1 -- Conn1/RConn1
  Three-Phase V-I Measurement1/RConn2 -- Conn2/RConn1
  Three-Phase V-I Measurement3/RConn1 -- Conn4/RConn1
  Three-Phase V-I Measurement3/RConn2 -- Conn5/RConn1

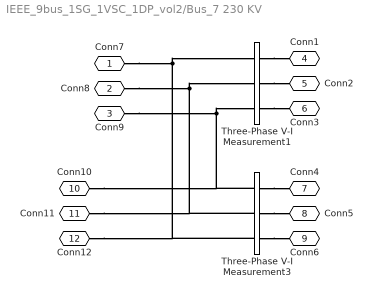
== system IEEE_9bus_1SG_1VSC_1DP_vol2/Bus_7 230 KV ==
  Three-Phase V-I Measurement1 : spsThreePhaseVIMeasurementLib/Three-Phase V-I Measurement  VoltageMeasurement=phase-to-ground  SetLabelV=on  LabelV=Vabc_7  Vpu=off  VpuLL=off  CurrentMeasurement=yes  SetLabelI=on  LabelI=Iabc_7  Ipu=off  Pbase=100e6  Vbase=230e3  OutputType=Complex  PhasorSimulation=off  PSBequivalent=0
  Three-Phase V-I Measurement3 : spsThreePhaseVIMeasurementLib/Three-Phase V-I Measurement  VoltageMeasurement=phase-to-ground  SetLabelV=on  LabelV=Vab  Vpu=off  VpuLL=off  CurrentMeasurement=yes  SetLabelI=on  LabelI=Iab  Ipu=off  Pbase=100e6  Vbase=230e3  OutputType=Complex  PhasorSimulation=off  PSBequivalent=0
  Conn7 : PMIOPort  Side=Left
  Conn8 : PMIOPort  Port=2  Side=Left
  Conn9 : PMIOPort  Port=3  Side=Left
  Conn1 : PMIOPort  Port=4  Side=Right
  Conn2 : PMIOPort  Port=5  Side=Right
  Conn3 : PMIOPort  Port=6  Side=Right
  Conn4 : PMIOPort  Port=7  Side=Right
  Conn5 : PMIOPort  Port=8  Side=Right
  Conn6 : PMIOPort  Port=9  Side=Right
  Conn10 : PMIOPort  Port=10  Side=Left
  Conn11 : PMIOPort  Port=11  Side=Left
  Conn12 : PMIOPort  Port=12  Side=Left
  connections:
  Three-Phase V-I Measurement3/RConn2 -- Conn5/RConn1
  Three-Phase V-I Measurement3/RConn1 -- Conn4/RConn1
  Three-Phase V-I Measurement1/RConn2 -- Conn2/RConn1
  Three-Phase V-I Measurement1/RConn1 -- Conn1/RConn1
  Three-Phase V-I Measurement1/RConn3 -- Conn3/RConn1
  Three-Phase V-I Measurement3/RConn3 -- Conn6/RConn1
  Conn7/RConn1 -- Three-Phase V-I Measurement3/LConn3 -- Conn12/RConn1 -- Three-Phase V-I Measurement1/LConn1
  Conn8/RConn1 -- Three-Phase V-I Measurement3/LConn2 -- Conn11/RConn1 -- Three-Phase V-I Measurement1/LConn2
  Conn9/RConn1 -- Conn10/RConn1 -- Three-Phase V-I Measurement3/LConn1 -- Three-Phase V-I Measurement1/LConn3

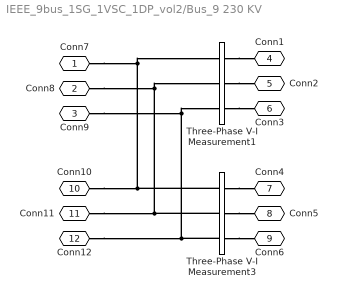
== system IEEE_9bus_1SG_1VSC_1DP_vol2/Bus_9 230 KV ==
  Three-Phase V-I Measurement1 : spsThreePhaseVIMeasurementLib/Three-Phase V-I Measurement  VoltageMeasurement=phase-to-ground  SetLabelV=on  LabelV=Vabc_9  Vpu=off  VpuLL=off  CurrentMeasurement=yes  SetLabelI=on  LabelI=Iabc_9  Ipu=off  Pbase=100e6  Vbase=230e3  OutputType=Complex  PhasorSimulation=off  PSBequivalent=0
  Three-Phase V-I Measurement3 : spsThreePhaseVIMeasurementLib/Three-Phase V-I Measurement  VoltageMeasurement=phase-to-ground  SetLabelV=on  LabelV=Vabc  Vpu=off  VpuLL=off  CurrentMeasurement=yes  SetLabelI=on  LabelI=Iabc  Ipu=off  Pbase=100e6  Vbase=230e3  OutputType=Complex  PhasorSimulation=off  PSBequivalent=0
  Conn7 : PMIOPort  Side=Left
  Conn8 : PMIOPort  Port=2  Side=Left
  Conn9 : PMIOPort  Port=3  Side=Left
  Conn1 : PMIOPort  Port=4  Side=Right
  Conn2 : PMIOPort  Port=5  Side=Right
  Conn3 : PMIOPort  Port=6  Side=Right
  Conn4 : PMIOPort  Port=7  Side=Right
  Conn5 : PMIOPort  Port=8  Side=Right
  Conn6 : PMIOPort  Port=9  Side=Right
  Conn10 : PMIOPort  Port=10  Side=Left
  Conn11 : PMIOPort  Port=11  Side=Left
  Conn12 : PMIOPort  Port=12  Side=Left
  connections:
  Conn12/RConn1 -- Three-Phase V-I Measurement3/LConn3 -- Conn9/RConn1 -- Three-Phase V-I Measurement1/LConn3
  Conn11/RConn1 -- Three-Phase V-I Measurement3/LConn2 -- Conn8/RConn1 -- Three-Phase V-I Measurement1/LConn2
  Conn10/RConn1 -- Three-Phase V-I Measurement3/LConn1 -- Conn7/RConn1 -- Three-Phase V-I Measurement1/LConn1
  Three-Phase V-I Measurement3/RConn3 -- Conn6/RConn1
  Three-Phase V-I Measurement1/RConn3 -- Conn3/RConn1
  Three-Phase V-I Measurement1/RConn1 -- Conn1/RConn1
  Three-Phase V-I Measurement1/RConn2 -- Conn2/RConn1
  Three-Phase V-I Measurement3/RConn1 -- Conn4/RConn1
  Three-Phase V-I Measurement3/RConn2 -- Conn5/RConn1

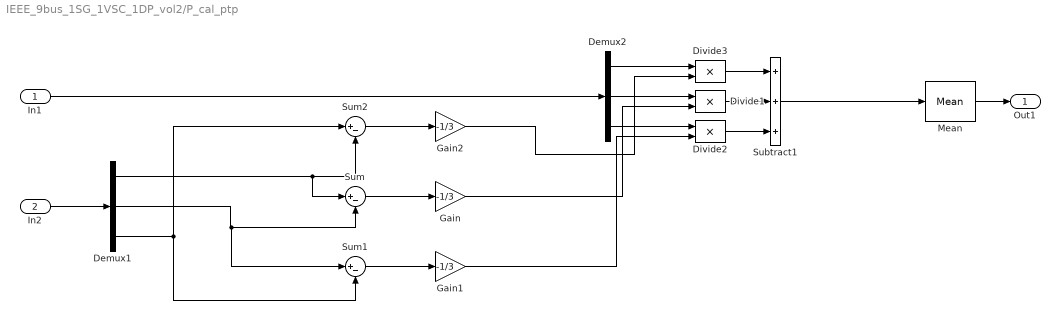
== system IEEE_9bus_1SG_1VSC_1DP_vol2/P_cal_ptp ==
  In1 : Inport
  In2 : Inport  Port=2
  Demux1 : Demux  Outputs=3
  Demux2 : Demux  Outputs=3
  Divide1 : Product  Inputs=**
  Divide2 : Product  Inputs=**
  Divide3 : Product  Inputs=**
  Gain : Gain  Gain=-1/3
  Gain1 : Gain  Gain=-1/3
  Gain2 : Gain  Gain=-1/3
  Mean : spsMeanLib/Mean  Freq=60  Vinit=1.636e8  Ts=0
  Subtract1 : Sum  Inputs=+++
  Sum : Sum  Inputs=|+-
  Sum1 : Sum  Inputs=|+-
  Sum2 : Sum  Inputs=|+-
  Out1 : Outport
  wires:
  Sum2/1 -> Gain2/1
  Demux1/3 -> Sum2/1, Sum1/2
  Demux1/1 -> Sum2/2, Sum/1
  Demux1/2 -> Sum1/1, Sum/2
  Demux2/2 -> Divide1/1
  Gain1/1 -> Divide2/2
  Divide1/1 -> Subtract1/2
  Divide3/1 -> Subtract1/1
  Sum1/1 -> Gain1/1
  In1/1 -> Demux2/1
  Divide2/1 -> Subtract1/3
  Demux2/3 -> Divide2/1
  Demux2/1 -> Divide3/1
  Gain/1 -> Divide1/2
  Sum/1 -> Gain/1
  Gain2/1 -> Divide3/2
  In2/1 -> Demux1/1
  Mean/1 -> Out1/1
  Subtract1/1 -> Mean/1

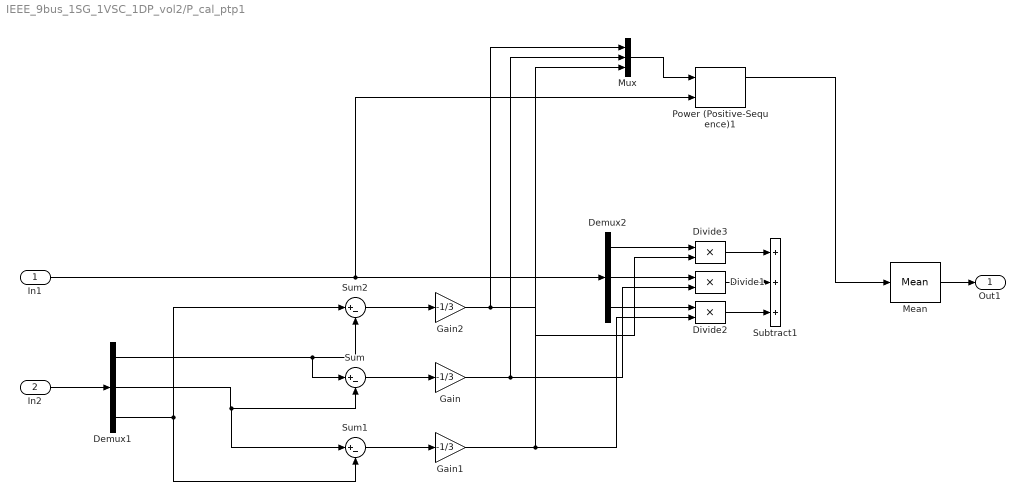
== system IEEE_9bus_1SG_1VSC_1DP_vol2/P_cal_ptp1 ==
  In1 : Inport
  In2 : Inport  Port=2
  Demux1 : Demux  Outputs=3
  Demux2 : Demux  Outputs=3
  Divide1 : Product  Inputs=**
  Divide2 : Product  Inputs=**
  Divide3 : Product  Inputs=**
  Gain : Gain  Gain=-1/3
  Gain1 : Gain  Gain=-1/3
  Gain2 : Gain  Gain=-1/3
  Mean : spsMeanLib/Mean  Freq=60  Vinit=(0.8553e8)  Ts=0
  Mux : Mux  Inputs=3
  Power (Positive-Sequence)1 : spsPowerPositiveSequenceLib/Power (Positive-Sequence)  Freq=60  Vinit=[0, 0]  Iinit=[0, 0]  Ts=1e-4
  Subtract1 : Sum  Inputs=+++
  Sum : Sum  Inputs=|+-
  Sum1 : Sum  Inputs=|+-
  Sum2 : Sum  Inputs=|+-
  Out1 : Outport
  wires:
  Sum2/1 -> Gain2/1
  Demux1/3 -> Sum2/1, Sum1/2
  Demux1/1 -> Sum2/2, Sum/1
  Demux1/2 -> Sum1/1, Sum/2
  Demux2/2 -> Divide1/1
  Gain1/1 -> Divide2/2, Mux/3
  Divide1/1 -> Subtract1/2
  Divide3/1 -> Subtract1/1
  Sum1/1 -> Gain1/1
  In1/1 -> Power (Positive-Sequence)1/2, Demux2/1
  Divide2/1 -> Subtract1/3
  Demux2/3 -> Divide2/1
  Demux2/1 -> Divide3/1
  Gain/1 -> Mux/2, Divide1/2
  Sum/1 -> Gain/1
  Gain2/1 -> Mux/1, Divide3/2
  In2/1 -> Demux1/1
  Mean/1 -> Out1/1
  Mux/1 -> Power (Positive-Sequence)1/1
  Power (Positive-Sequence)1/1 -> Mean/1

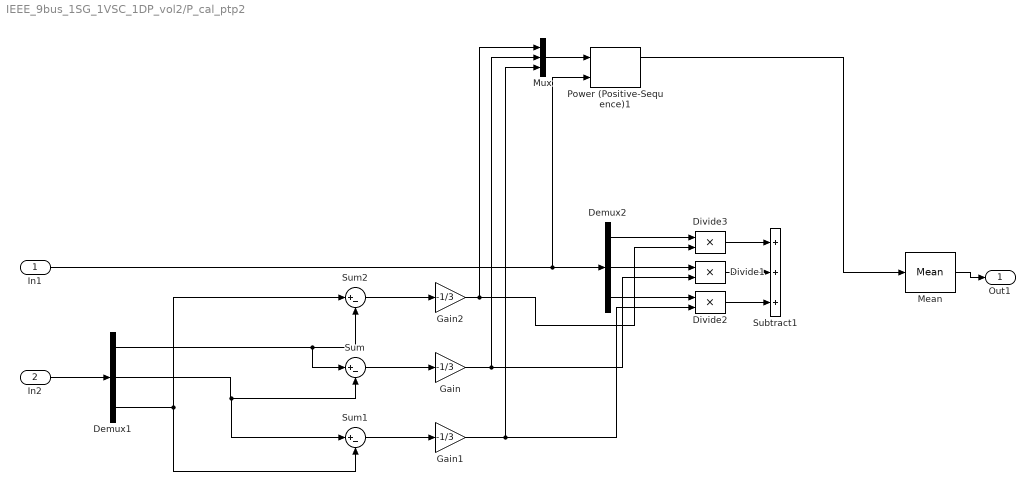
== system IEEE_9bus_1SG_1VSC_1DP_vol2/P_cal_ptp2 ==
  In1 : Inport
  In2 : Inport  Port=2
  Demux1 : Demux  Outputs=3
  Demux2 : Demux  Outputs=3
  Divide1 : Product  Inputs=**
  Divide2 : Product  Inputs=**
  Divide3 : Product  Inputs=**
  Gain : Gain  Gain=-1/3
  Gain1 : Gain  Gain=-1/3
  Gain2 : Gain  Gain=-1/3
  Mean : spsMeanLib/Mean  Freq=60  Vinit=(0.7317e8)  Ts=0
  Mux : Mux  Inputs=3
  Power (Positive-Sequence)1 : spsPowerPositiveSequenceLib/Power (Positive-Sequence)  Freq=60  Vinit=[0, 0]  Iinit=[0, 0]  Ts=1e-4
  Subtract1 : Sum  Inputs=+++
  Sum : Sum  Inputs=|+-
  Sum1 : Sum  Inputs=|+-
  Sum2 : Sum  Inputs=|+-
  Out1 : Outport
  wires:
  Sum2/1 -> Gain2/1
  Demux1/3 -> Sum2/1, Sum1/2
  Demux1/1 -> Sum2/2, Sum/1
  Demux1/2 -> Sum1/1, Sum/2
  Demux2/2 -> Divide1/1
  Gain1/1 -> Mux/3, Divide2/2
  Divide1/1 -> Subtract1/2
  Divide3/1 -> Subtract1/1
  Sum1/1 -> Gain1/1
  In1/1 -> Power (Positive-Sequence)1/2, Demux2/1
  Divide2/1 -> Subtract1/3
  Demux2/3 -> Divide2/1
  Demux2/1 -> Divide3/1
  Gain/1 -> Mux/2, Divide1/2
  Sum/1 -> Gain/1
  Gain2/1 -> Mux/1, Divide3/2
  In2/1 -> Demux1/1
  Mean/1 -> Out1/1
  Mux/1 -> Power (Positive-Sequence)1/1
  Power (Positive-Sequence)1/1 -> Mean/1

== system IEEE_9bus_1SG_1VSC_1DP_vol2/Subsystem ==
  cte1 : Constant
  cte2 : Constant  Value=2
  cte3 : Constant  Value=0
  Generic : Outport  VectorParamsAs1DForOutWhenUnconnected=off
  Multiband : Outport  Port=2  VectorParamsAs1DForOutWhenUnconnected=off
  No PSS : Outport  Port=3  VectorParamsAs1DForOutWhenUnconnected=off
  wires:
  cte1/1 -> Generic/1
  cte2/1 -> Multiband/1
  cte3/1 -> No PSS/1
